simulink model "H175_Anode_Integration"  (R2023a)
settings: Solver=VariableStepAuto  StartTime=0.0  StopTime=80  RelTol=1e-3
values from neighbouring files (symbols this model uses):
  anode_tube_D = 0.01    [All_Properties.mat]    (also in anode_subsystem_parameters.m; environment_parameters.m)
  D = 0.01    [All_Properties.mat]    (also in anode_subsystem_parameters.m)
  densityHydrogen = 0.0899    [All_Properties.mat]    (also in Valve_Init.m; anode_subsystem_parameters.m)
  Kv_VL6112 = 0.8    [All_Properties.mat]    (also in anode_subsystem_parameters.m)
  N2_T = [-56.55 -50 -40 -30 -20 -10 -5 -4 -3 -2 -1 0 ... (52 elements, 1x52)]    [All_Properties.mat]    (also in anode_subsystem_parameters.m = [-56.55 -50 -40 -30 -20 -10 -5 -4 -3 -2 -1 0 1 2 3 4 5 10 20; environment_parameters.m = [-56.55, -50:10:-10, -5:1:5, 10:10:350]; stack_model_harness_parameters.m = [-56.55, -50:10:-10, -5:1:5, 10:10:350])
  p_range = 0.005    [All_Properties.mat]    (also in anode_subsystem_parameters.m)
  r_max = 0.2    [All_Properties.mat]    (also in anode_subsystem_parameters.m)
  r_min = 0.0001    [All_Properties.mat]    (also in anode_subsystem_parameters.m)
  responseTimeValve = 0.013    [All_Properties.mat]    (also in anode_subsystem_parameters.m)
libraries: fl_lib x75, nesl_utility x39, SimscapeFluids_lib x1
(part 1 of 2)
settings Model: Creator=debjani.ghosh  LastModifiedBy=adrian.taveras
settings DataIOCC: SaveFormat=StructureWithTime  ReturnWorkspaceOutputs=off  LoggingToFile=on
settings SimscapeCC: SimscapeLogType=all  SimscapeLogOpenViewer=on  SimscapeLogLimitData=off

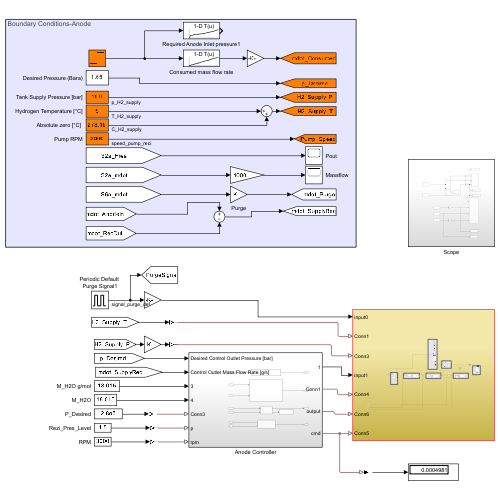
[thumbnail: Simulink's stored preview of the top-level diagram]
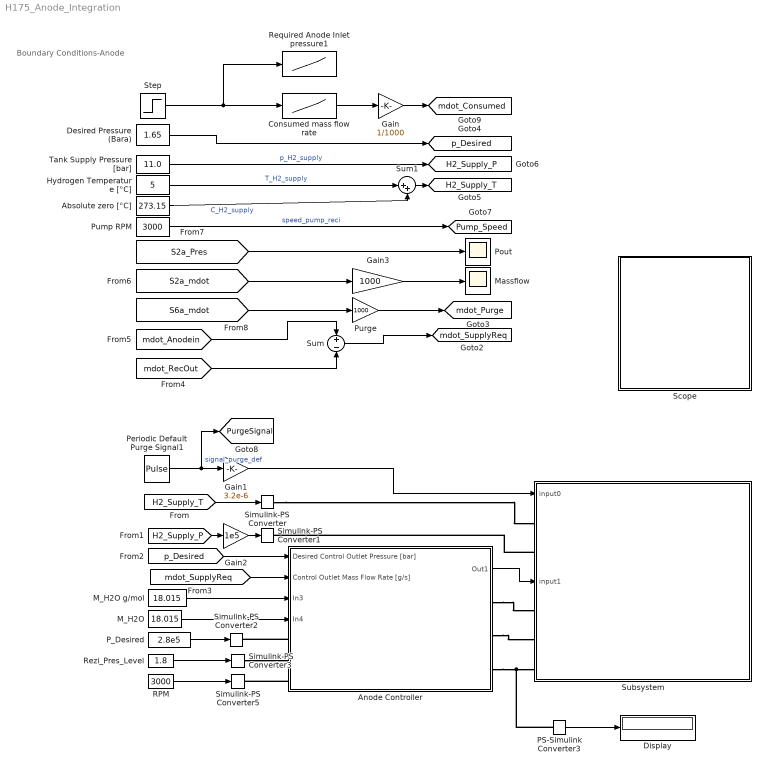
== system H175_Anode_Integration ==
  note: Boundary Conditions-Anode
  "Absolute zero [°C] " : Constant  Value=273.15
  Anode Controller : Subsystem
  Consumed mass flow rate : Lookup_n-D  NumberOfTableDimensions=1  BreakpointsForDimension1=[0;20;100;200;300;400;500;600]  Table=[0;0.1;0.5;1;1.5;2;2.5;3]  InternalRulePriority=Speed  RndMeth=Simplest
  Desired Pressure (Bara) : Constant  Value=1.65
  Display : Display
  Gain : Gain  Gain=1/1000
  Gain1 : Gain  Gain=3.2e-6
  Gain2 : Gain  Gain=1e5
  Gain3 : Gain  Gain=1000
  Hydrogen Temperature [°C] : Constant  Value=5
  M_H2O : Constant  Value=18.015
  M_H2O g/mol : Constant  Value=18.015
  Massflow : Scope
  PS-Simulink Converter3 : nesl_utility/PS-Simulink Converter  PhysicalDomain=network_engine_domain  SubClassName=ps_output  LeftPortType=input  RightPortType=output  PseudoPeriodic=off  Frequencies=[]  VectorFormat=inherit  Unit=inherit  AffineConversion=off
  P_Desired : Constant  Value=2.8e5
  Periodic Default Purge Signal1 : DiscretePulseGenerator  PulseType=Time based  Period=3  PulseWidth=5
  Pout : Scope
  Pump RPM : Constant  Value=3000
  Purge : Gain  Gain=1000
  RPM : Constant  Value=3000
  Required Anode Inlet pressure1 : Lookup_n-D  NumberOfTableDimensions=1  BreakpointsForDimension1=[0;20;100;200;300;400;500;600]  Table=[1;1.4;1.6;1.7;1.8;2;2.3;2.6]  InternalRulePriority=Speed  RndMeth=Simplest
  Rezi_Pres_Level : Constant  Value=1.8
  Scope : Subsystem
  Simulink-PS Converter : nesl_utility/Simulink-PS Converter  PhysicalDomain=network_engine_domain  SubClassName=ps_input  LeftPortType=input  RightPortType=output  PseudoPeriodic=off  Frequencies=[]  NoiseDistribution=none  NoiseParameters=[]  Unit=K  AffineConversion=off  FilteringAndDerivatives=provide  SimscapeFilterOrder=1  InputFilterTimeConstant=0.001  UdotUserProvided=0
  Simulink-PS Converter1 : nesl_utility/Simulink-PS Converter  PhysicalDomain=network_engine_domain  SubClassName=ps_input  LeftPortType=input  RightPortType=output  PseudoPeriodic=off  Frequencies=[]  NoiseDistribution=none  NoiseParameters=[]  Unit=Pa  AffineConversion=off  FilteringAndDerivatives=provide  SimscapeFilterOrder=1  InputFilterTimeConstant=0.001  UdotUserProvided=0
  Simulink-PS Converter2 : nesl_utility/Simulink-PS Converter  PhysicalDomain=network_engine_domain  SubClassName=ps_input  LeftPortType=input  RightPortType=output  PseudoPeriodic=off  Frequencies=[]  NoiseDistribution=none  NoiseParameters=[]  Unit=1  AffineConversion=off  FilteringAndDerivatives=provide  SimscapeFilterOrder=1  InputFilterTimeConstant=0.001  UdotUserProvided=0
  Simulink-PS Converter3 : nesl_utility/Simulink-PS Converter  PhysicalDomain=network_engine_domain  SubClassName=ps_input  LeftPortType=input  RightPortType=output  PseudoPeriodic=off  Frequencies=[]  NoiseDistribution=none  NoiseParameters=[]  Unit=1  AffineConversion=off  FilteringAndDerivatives=provide  SimscapeFilterOrder=1  InputFilterTimeConstant=0.001  UdotUserProvided=0
  Simulink-PS Converter5 : nesl_utility/Simulink-PS Converter  PhysicalDomain=network_engine_domain  SubClassName=ps_input  LeftPortType=input  RightPortType=output  PseudoPeriodic=off  Frequencies=[]  NoiseDistribution=none  NoiseParameters=[]  Unit=1  AffineConversion=off  FilteringAndDerivatives=provide  SimscapeFilterOrder=1  InputFilterTimeConstant=0.001  UdotUserProvided=0
  Step : Step  Time=40  Before=200  After=350  SampleTime=0
  Subsystem : Subsystem
      settings: PortSchema="{\"entries\":[{\"content\":{\"sides\":[{\"content\":{\"connectorIds\":[\"In1\",\"LConn1\",\"LConn2\",\"In2\",\"LConn3\",\"LConn4\",\"LConn5\"]},\"type\":\"ConnectorPlacement.EquallySpacedRectSide\",\"uuid\":\"6d276737-1cfb-43f0-89a6-ca57f89f04f9\"},{\"content\":{\"side\":\"RIGHT\"},\"type\":\"ConnectorPlacement.EquallySpacedRectSide\",\"uuid\":\"f7ce7b2b-f458-4a7d-a84b-f12d4a9a3d73\"},{\"content\":{\"side\":\"TOP\"},\"type\":\"ConnectorPlacement.EquallySpacedRectSide\",\"uuid\":\"f2759a84-f209-4626-aa5e-b52256180764\"}]},\"type\":\"ConnectorPlacement.EquallySpacedConnector\",\"uuid\":\"a55dce8e-c3c8-40fa-9a6a-dcd78737938e\"}],\"packageUris\":[\"http://schema.mathworks.com/mf0/Connector/R2020b\"],\"version\":\"1.0\"}"
  Sum : Sum  Inputs=+-
  Sum1 : Sum  Inputs=|++
  Tank Supply Pressure [bar] : Constant  Value=11.0
  tag scope: H2_Supply_P=global, H2_Supply_T=global, Pump_Speed=global, PurgeSignal=global, mdot_Consumed=global, mdot_Purge=global, mdot_SupplyReq=global, p_Desired=global
  wires:
  Consumed mass flow rate/1 -> Gain/1
  Hydrogen Temperature [°C]/1 -> Sum1/1  "T_H2_supply"
  "Absolute zero [°C] "/1 -> Sum1/2  "C_H2_supply"
  Sum1/1 -> [H2_Supply_T]
  Tank Supply Pressure [bar]/1 -> [H2_Supply_P]  "p_H2_supply"
  Pump RPM/1 -> [Pump_Speed]  "speed_pump_reci"
  Gain/1 -> [mdot_Consumed]
  Desired Pressure (Bara)/1 -> [p_Desired]
  Step/1 -> Required Anode Inlet pressure1/1, Consumed mass flow rate/1
  Gain2/1 -> Simulink-PS Converter1/1
  [H2_Supply_P] -> Gain2/1
  [H2_Supply_T] -> Simulink-PS Converter/1
  P_Desired/1 -> Simulink-PS Converter2/1
  Gain3/1 -> Massflow/1
  [S2a_mdot] -> Gain3/1
  [S2a_Pres] -> Pout/1
  Sum/1 -> [mdot_SupplyReq]
  [mdot_Anodein] -> Sum/1
  [mdot_RecOut] -> Sum/2
  Rezi_Pres_Level/1 -> Simulink-PS Converter3/1
  PS-Simulink Converter3/1 -> Display/1
  RPM/1 -> Simulink-PS Converter5/1
  Periodic Default Purge Signal1/1 -> Gain1/1, [PurgeSignal]  "signal_purge_def"
  Purge/1 -> [mdot_Purge]
  [S6a_mdot] -> Purge/1
  [p_Desired] -> Anode Controller/1(Desired Control Outlet Pressure [bar])
  [mdot_SupplyReq] -> Anode Controller/2(Control Outlet Mass Flow Rate [g/s])
  M_H2O g/mol/1 -> Anode Controller/3(In3)
  M_H2O/1 -> Anode Controller/4(In4)
  Gain1/1 -> Subsystem/1(input0)
  Anode Controller/1(Out1) -> Subsystem/2(input1)
  connections:
  PS-Simulink Converter3/LConn1 -- Anode Controller/RConn3 -- Subsystem/LConn5
  Anode Controller/LConn1 -- Simulink-PS Converter2/RConn1
  Simulink-PS Converter3/RConn1 -- Anode Controller/LConn2
  Anode Controller/LConn3 -- Simulink-PS Converter5/RConn1
  Simulink-PS Converter/RConn1 -- Subsystem/LConn1
  Subsystem/LConn2 -- Simulink-PS Converter1/RConn1
  Anode Controller/RConn1 -- Subsystem/LConn3
  Anode Controller/RConn2 -- Subsystem/LConn4

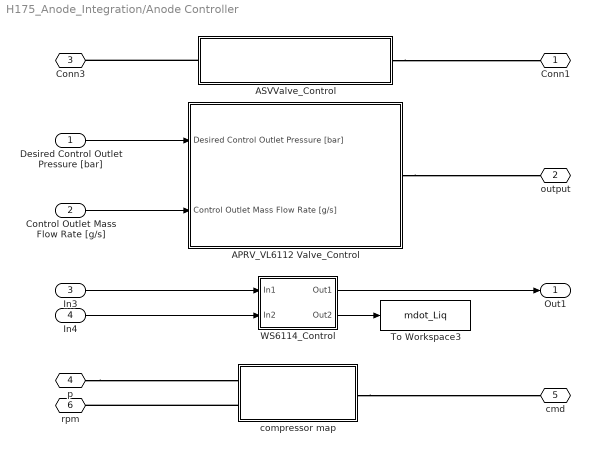
== system H175_Anode_Integration/Anode Controller ==
  Desired Control Outlet Pressure [bar] : Inport
  Control Outlet Mass Flow Rate [g/s] : Inport  Port=2
  In3 : Inport  Port=3
  In4 : Inport  Port=4
  APRV_VL6112 Valve_Control : Subsystem
  ASVValve_Control : Subsystem
  To Workspace3 : ToWorkspace  VariableName=mdot_Liq  SaveFormat=Structure With Time  SampleTime=-1
  WS6114_Control : Subsystem
  compressor map : Subsystem
  Conn1 : PMIOPort  Side=Right
  output : PMIOPort  Port=2  Side=Right
  Conn3 : PMIOPort  Port=3  Side=Left
  p : PMIOPort  Port=4  Side=Left
  cmd : PMIOPort  Port=5  Side=Right
  rpm : PMIOPort  Port=6  Side=Left
  Out1 : Outport
  wires:
  Control Outlet Mass Flow Rate [g/s]/1 -> APRV_VL6112 Valve_Control/2(Control Outlet Mass Flow Rate [g/s])
  WS6114_Control/1(Out1) -> Out1/1
  Desired Control Outlet Pressure [bar]/1 -> APRV_VL6112 Valve_Control/1(Desired Control Outlet Pressure [bar])
  WS6114_Control/2(Out2) -> To Workspace3/1
  In3/1 -> WS6114_Control/1(In1)
  In4/1 -> WS6114_Control/2(In2)
  connections:
  p/RConn1 -- compressor map/LConn1
  ASVValve_Control/RConn1 -- Conn1/RConn1
  compressor map/RConn1 -- cmd/RConn1
  ASVValve_Control/LConn1 -- Conn3/RConn1
  compressor map/LConn2 -- rpm/RConn1
  APRV_VL6112 Valve_Control/RConn1 -- output/RConn1

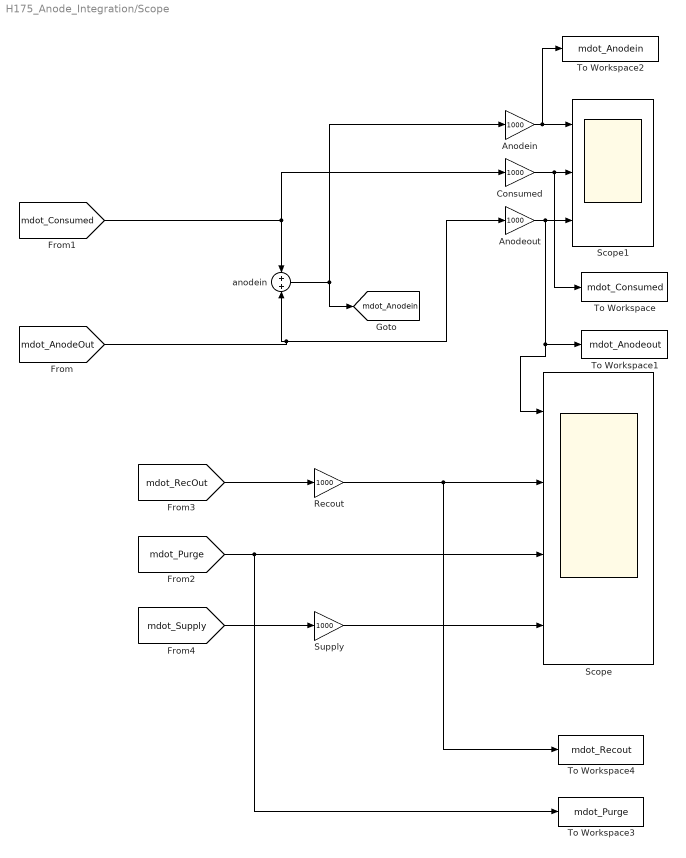
== system H175_Anode_Integration/Scope ==
  Anodein : Gain  Gain=1000
  Anodeout : Gain  Gain=1000
  Consumed : Gain  Gain=1000
  Recout : Gain  Gain=1000
  Scope : Scope  NumInputPorts=4
  Scope1 : Scope  NumInputPorts=3
  Supply : Gain  Gain=1000
  To Workspace : ToWorkspace  VariableName=mdot_Consumed  SaveFormat=Structure With Time  SampleTime=-1
  To Workspace1 : ToWorkspace  VariableName=mdot_Anodeout  SaveFormat=Structure With Time  SampleTime=-1
  To Workspace2 : ToWorkspace  VariableName=mdot_Anodein  SaveFormat=Structure With Time  SampleTime=-1
  To Workspace3 : ToWorkspace  VariableName=mdot_Purge  SaveFormat=Structure With Time  SampleTime=-1
  To Workspace4 : ToWorkspace  VariableName=mdot_Recout  SaveFormat=Structure With Time  SampleTime=-1
  anodein : Sum
  tag scope: mdot_Anodein=global
  wires:
  [mdot_Consumed] -> anodein/1, Consumed/1
  [mdot_AnodeOut] -> Anodeout/1, anodein/2
  Anodein/1 -> To Workspace2/1, Scope1/1
  Anodeout/1 -> Scope/1, To Workspace1/1, Scope1/3
  Consumed/1 -> To Workspace/1, Scope1/2
  [mdot_Purge] -> To Workspace3/1, Scope/3
  anodein/1 -> [mdot_Anodein], Anodein/1
  Recout/1 -> To Workspace4/1, Scope/2
  [mdot_RecOut] -> Recout/1
  [mdot_Supply] -> Supply/1
  Supply/1 -> Scope/4

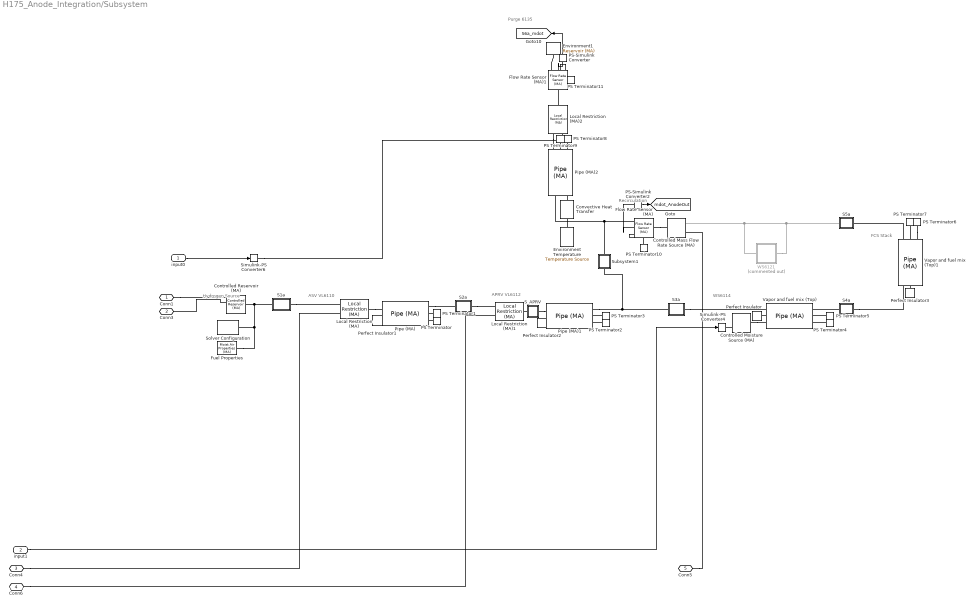
== system H175_Anode_Integration/Subsystem ==
  note: Purge 6135
  note: FCS Stack
  note: Recirculation
  note: WS6114
  note: APRV VL6112
  note: ASV VL6110
  note: Hydrogen Source
  input0 : Inport
  input1 : Inport  Port=2
  " WS6121" : Subsystem  Tag=PublishSubsystem  Commented=on
  Controlled Mass Flow Rate Source (MA) : fl_lib/Moist Air/Sources/Controlled Mass Flow Rate Source (MA)  power_spec=foundation.enum.power_spec.isentropic  area_A=pi*anode_tube_D^2/4 m^2  area_B=pi*anode_tube_D^2/4 m^2
      settings: InternalSimscapePortConfiguration="{\"Bottom\":[],\"Left\":[{\"id\":\"A\",\"label\":\"A\",\"type\":\"foundation.moist_air.moist_air\"},{\"id\":\"M\",\"label\":\"M\",\"type\":\"input\"}],\"Right\":[{\"id\":\"B\",\"label\":\"B\",\"type\":\"foundation.moist_air.moist_air\"}],\"Top\":[]}"
  Controlled Moisture Source (MA) : fl_lib/Moist Air/Sources/Moisture & Trace Gas Sources/Controlled Moisture Source (MA)  moisture_source_spec=foundation.enum.moisture_source_spec.liquid  Phi_S_specify=off  Phi_S_priority=None  Phi_S=0 kW  Phi_S_nominal_specify=off  Phi_S_nominal_unit=kW  Phi_S_nominal_value=1  mdot_w_S_specify=off  mdot_w_S_priority=None  mdot_w_S=0 kg/s  mdot_w_S_nominal_specify=off  mdot_w_S_nominal_unit=kg/s  mdot_w_S_nominal_value=1
      settings: InternalSimscapePortConfiguration="{\"Bottom\":[],\"Left\":[{\"id\":\"S\",\"label\":\"S\",\"type\":\"foundation.moist_air.moist_air_source\"}],\"Right\":[{\"id\":\"M\",\"label\":\"M\",\"type\":\"input\"},{\"id\":\"T\",\"label\":\"T\",\"type\":\"input\"}],\"Top\":[]}"
  Controlled Reservoir (MA) : fl_lib/Moist Air/Elements/Controlled Reservoir (MA)  moisture_spec=foundation.enum.moistureSpec.RelativeHumidity  trace_gas_spec=foundation.enum.trace_gas_spec.mass_fraction  RH_ws=1  area_A=0.01 m^2  input_error_spec=foundation.enum.input_range_error.warn
      settings: InternalSimscapePortConfiguration="{\"Bottom\":[],\"Left\":[{\"id\":\"A\",\"label\":\"A\",\"type\":\"foundation.moist_air.moist_air\"}],\"Right\":[{\"id\":\"T\",\"label\":\"T\",\"type\":\"input\"},{\"id\":\"P\",\"label\":\"P\",\"type\":\"input\"},{\"id\":\"W\",\"label\":\"W\",\"type\":\"input\"},{\"id\":\"G\",\"label\":\"G\",\"type\":\"input\"}],\"Top\":[]}"
  Convective Heat Transfer : fl_lib/Thermal/Thermal Elements/Convective Heat Transfer  thermal_type=foundation.enum.constant_variable.constant  area=pi*anode_tube_D*1 m^2  heat_tr_coeff=20 W/(m^2 * K)  min_heat_tr_coeff=1e-3 W/(K*m^2)  T_specify=off  T_priority=None  T=0 K  T_nominal_specify=off  T_nominal_unit=K  T_nominal_value=1  Q_specify=off  Q_priority=None  Q=0 W  Q_nominal_specify=off  Q_nominal_unit=W  Q_nominal_value=1
  Environment Temperature : fl_lib/Thermal/Thermal Sources/Temperature Source  temperature=env_T degC
  Environment1 : fl_lib/Moist Air/Elements/Reservoir (MA)  pressure_spec=foundation.enum.pressure_spec.atmospheric  reservoir_pressure=0.101325 MPa  temperature_spec=foundation.enum.temperature_spec.atmospheric  reservoir_temperature=293.15 K  moisture_spec=foundation.enum.moistureSpec.RelativeHumidity  reservoir_RH=0.5  reservoir_x_w=0.01  reservoir_y_w=0.01  reservoir_HR=0.01  reservoir_Tw=287 K  trace_gas_spec=foundation.enum.trace_gas_spec.mass_fraction  reservoir_x_g=0.001  reservoir_y_g=0.001  RH_ws=1  area_A=0.01 m^2
  Flow Rate Sensor (MA) : fl_lib/Moist Air/Sensors/Flow Rate Sensor (MA)  mass_flow_measure=true  volumetric_flow_measure=false  volumetric_flow_conditions=foundation.enum.volumetric_flow_conditions.actual  p_std=0.101325 MPa  T_std=20 degC  RH_std=0.65  energy_flow_measure=true  vapor_flow_measure=false  gas_flow_measure=false
      settings: InternalSimscapePortConfiguration="{\"Bottom\":[{\"id\":\"PHI\",\"label\":\"φ\",\"type\":\"output\"}],\"Left\":[{\"id\":\"A\",\"label\":\"A\",\"type\":\"foundation.moist_air.moist_air\"}],\"Right\":[{\"id\":\"B\",\"label\":\"B\",\"type\":\"foundation.moist_air.moist_air\"},{\"id\":\"M\",\"label\":\"M\",\"type\":\"output\"}],\"Top\":[]}"
  Flow Rate Sensor (MA)1 : fl_lib/Moist Air/Sensors/Flow Rate Sensor (MA)  mass_flow_measure=true  volumetric_flow_measure=false  volumetric_flow_conditions=foundation.enum.volumetric_flow_conditions.actual  p_std=0.101325 MPa  T_std=20 degC  RH_std=0.65  energy_flow_measure=true  vapor_flow_measure=false  gas_flow_measure=false
      settings: InternalSimscapePortConfiguration="{\"Bottom\":[{\"id\":\"PHI\",\"label\":\"φ\",\"type\":\"output\"}],\"Left\":[{\"id\":\"A\",\"label\":\"A\",\"type\":\"foundation.moist_air.moist_air\"}],\"Right\":[{\"id\":\"B\",\"label\":\"B\",\"type\":\"foundation.moist_air.moist_air\"},{\"id\":\"M\",\"label\":\"M\",\"type\":\"output\"}],\"Top\":[]}"
  Fuel Properties : fl_lib/Moist Air/Utilities/Moist Air Properties (MA)  R_a=N2_R J/kg/K  T_TLU=N2_T degC  h_a_TLU=N2_h kJ/kg  mu_a_TLU=N2_mu s*uPa  k_a_TLU=N2_k mW/m/K  p_min=1 kPa  p_max=inf MPa  T_min=min(N2_T) degC  T_max=max(N2_T) degC  properties_range_check=simscape.enum.assert.action.error  p_atm=0.101325 MPa  T_atm=20 degC  R_w=461.523 J/kg/K  p_ws_TLU=[1.71168953425982e-06; 3.93770601979424e-06; 1.28411717710344e-05; 3.80051394873809e-05; .00010323902900209; .000259873810798063; .000401741022116384; .000437454836117844; .000476040820618202; .000517704666185737; .000562664883741207; .000611212677444345; .000657088049117899; .000705987905898279; .000758082381149132; .000813549384183233; .000872574861129522; .00122818386934022; .0023392147667769; .00424668834054807; .00738442748706953; .0123512704340234; .0199458019246787; .0312006356960619; .0474147199263783; .0701823607447713; .10141797792131; .143375967241115; .198665399739302; .270259606559999; .361500961984849; .476101381081492; .618139196722055; .792053183687694; 1.0026345688121; 1.25501792086105; 1.55467186826983; 1.90739066433297; 2.31928772772542; 2.79679245576864; 3.34665187151016; 3.97593907083533; 4.69207105435535; 5.5028394740883; 6.41645928168037; 7.4416425436169; 8.58770832955728; 9.86474556030261; 11.2838558865497; 12.8575218898034; 14.6001810568052; 16.5291642526045] MPa  h_w_vap_TLU=[2836.88241275372; 2837.81392500514; 2838.63937175807; 2838.7309929628; 2838.06905313927; 2836.62597341095; 2835.60023952573; 2835.37006381376; 2835.13143158077; 2834.88429145066; 2834.62859062897; 2500.93420564316; 2498.55329907119; 2496.17495082036; 2493.79885912205; 2491.42474723191; 2489.05236104642; 2477.20875029194; 2453.54955988604; 2429.83856603313; 2406.00136954922; 2381.97406342174; 2357.69101156389; 2333.08088387814; 2308.06565480412; 2282.56034405021; 2256.47287422313; 2229.70428017508; 2202.14968030993; 2173.69998896199; 2144.24368406447; 2113.66758247452; 2081.85585110571; 2048.68725710494; 2014.03141249899; 1977.7449923284; 1939.66849592886; 1899.62342931686; 1857.40930169838; 1812.79975416601; 1765.53721731251; 1715.32525772152; 1661.81700477787; 1604.59703745016; 1543.1534616334; 1476.83692476464; 1404.80240352424; 1325.92091736114; 1238.61667822208; 1140.5102987018; 1027.62017777647; 892.733785613825] kJ/kg  h_w_TLU=[2396.55944251649; 2408.68643343608; 2427.1988031141; 2445.702165897; 2464.18429108356; 2482.62529466839; 2491.82135326629; 2493.6580151792; 2495.49372578218; 2497.32843835745; 2499.16210446923; 2500.99462758899; 2502.83092214066; 2504.6665223621; 2506.50140563013; 2508.335548891; 2510.16892865793; 2519.32352241995; 2537.56068088674; 2555.67742615292; 2573.6403223998; 2591.4109179101; 2608.9455037701; 2626.19492016262; 2643.10444358428; 2659.61377634497; 2675.58278696023; 2696.1846256545; 2716.49989553741; 2736.6235210957; 2756.61216047011; 2776.50561773853; 2796.33378922508; 2816.11979583049; 2835.88181423877; 2855.63430574511; 2875.38889327595; 2895.15500577172; 2914.94035964689; 2934.75132290228; 2954.59319330244; 2974.47041285505; 2994.38673458964; 3014.34535328009; 3034.34900867103; 3054.40006755764; 3074.50058946898; 3094.65237953784; 3114.85703128106; 3135.11596137801; 3155.43043805905; 3175.80160435813] kJ/kg  mu_w_TLU=[6.81365662228272; 7.04953750742707; 7.40970098298307; 7.76991278093907; 8.13017290129507; 8.49048134405107; 8.67065368632907; 8.70668960445667; 8.74272600580827; 8.77876289038387; 8.81480025818347; 8.85083810920707; 8.88687644345467; 8.92291526092627; 8.95895456162187; 8.99499434554147; 9.03103461268507; 9.21124319676307; 9.57169660671907; 9.93219833907507; 10.2927483938311; 10.6533467709871; 11.0139934705431; 11.3746884924991; 11.7354318368551; 12.0962235036111; 12.4570634927671; 12.8179518043231; 13.1788884382791; 13.5398733946351; 13.9009066733911; 14.2619882745471; 14.6231181981031; 14.9842964440591; 15.3455230124151; 15.7067979031711; 16.0681211163271; 16.4294926518831; 16.7909125098391; 17.1523806901951; 17.5138971929511; 17.8754620181071; 18.2370751656631; 18.5987366356191; 18.9604464279751; 19.3222045427311; 19.6840109798871; 20.0458657394431; 20.4077688213991; 20.7697202257551; 21.1317199525111; 21.4937680016671] s*uPa  k_w_TLU=[11.46288215976; 11.941997488935; 12.676358586935; 13.414208884935; 14.155548382935; 14.900377080935; 15.274099879935; 15.348949115735; 15.423833243535; 15.498752263335; 15.573706175135; 15.648694978935; 15.723718674735; 15.798777262535; 15.873870742335; 15.948999114135; 16.024162377935; 16.400502076935; 17.155798374935; 17.914583872935; 18.676858570935; 19.442622468935; 20.211875566935; 20.984617864935; 21.760849362935; 22.540570060935; 23.323779958935; 24.110479056935; 24.900667354935; 25.694344852935; 26.491511550935; 27.292167448935; 28.096312546935; 28.903946844935; 29.715070342935; 30.529683040935; 31.347784938935; 32.169376036935; 32.994456334935; 33.823025832935; 34.655084530935; 35.490632428935; 36.329669526935; 37.172195824935; 38.018211322935; 38.867716020935; 39.720709918935; 40.577193016935; 41.437165314935; 42.300626812935; 43.167577510935; 44.038017408935] mW/m/K  D_w=25 mm^2/s  trace_gas_model=foundation.enum.trace_gas_model.track_properties  R_g=H2_R J/kg/K  h_g_TLU=H2_h kJ/kg  mu_g_TLU=H2_mu s*uPa  k_g_TLU=H2_k mW/m/K  D_g=H2_D mm^2/s
      settings: AttributesFormatString=|
      | dry air --> N2
      | water vapor --> H2O
      | trace gas --> H2
  Local Restriction (MA) : fl_lib/Moist Air/Elements/Local Restriction (MA)  restriction_type=foundation.enum.restriction_type.variable  restriction_area=0.005 m^2  min_area=0.00001e-6 m^2  max_area=4.75e-6 m^2  area=0.00358 m^2  Cd=0.80  B_lam=0.999
      settings: LogSimulationData=on
  Local Restriction (MA)1 : fl_lib/Moist Air/Elements/Local Restriction (MA)  restriction_type=foundation.enum.restriction_type.variable  restriction_area=0.005 m^2  min_area=0.00001e-6 m^2  max_area=4.75e-6 m^2  area=0.00358 m^2  Cd=0.80  B_lam=0.999
      settings: LogSimulationData=on
  Local Restriction (MA)2 : fl_lib/Moist Air/Elements/Local Restriction (MA)  restriction_type=foundation.enum.restriction_type.variable  restriction_area=0.005 m^2  min_area=0.00001e-6 m^2  max_area=3.2e-6 m^2  area=0.00358 m^2  Cd=0.80  B_lam=0.999
      settings: LogSimulationData=on
  PS Terminator{,1..11} (12 alike) : fl_lib/Physical Signals/Sinks/PS Terminator
  PS-Simulink Converter : nesl_utility/PS-Simulink Converter  PhysicalDomain=network_engine_domain  SubClassName=ps_output  LeftPortType=input  RightPortType=output  PseudoPeriodic=off  Frequencies=[]  VectorFormat=inherit  Unit=inherit  AffineConversion=off
  PS-Simulink Converter2 : nesl_utility/PS-Simulink Converter  PhysicalDomain=network_engine_domain  SubClassName=ps_output  LeftPortType=input  RightPortType=output  PseudoPeriodic=off  Frequencies=[]  VectorFormat=inherit  Unit=inherit  AffineConversion=off
  Perfect Insulator{,1..3} (4 alike) : fl_lib/Thermal/Thermal Elements/Perfect Insulator  T_specify=off  T_priority=None  T=0 K  T_nominal_specify=off  T_nominal_unit=K  T_nominal_value=1
  Pipe (MA) : fl_lib/Moist Air/Elements/Pipe (MA)  length=1 m  area=pi*anode_tube_D^2/4 m^2  Dh=anode_tube_D m  length_add=0.1 m  roughness=15e-6 m  Re_lam=2000  Re_tur=4000  shape_factor=64  Nu_lam=3.66  wall_condensation=simscape.enum.onoff.off  RH_ws=1  time_constant=1e-3 s  moisture_trace_gas_source=foundation.enum.moisture_trace_gas_source.none  moisture_source_spec=foundation.enum.moisture_source_spec.vapor  moisture_mass_flow=0 kg/s  moisture_temperature_spec=foundation.enum.temperature_spec.atmospheric  moisture_temperature=293.15 K  trace_gas_mass_flow=0 kg/s  trace_gas_temperature_spec=foundation.enum.temperature_spec.atmospheric  trace_gas_temperature=293.15 K  p_I_specify=on  p_I_priority=High  p_I=env_p MPa  p_I_nominal_specify=off  p_I_nominal_unit=MPa  p_I_nominal_value=1  T_I_specify=on  T_I_priority=High  T_I=env_T degC  T_I_nominal_specify=off  T_I_nominal_unit=K  T_I_nominal_value=1  RH_I_specify=off  RH_I_priority=High  RH_I=0  RH_I_nominal_specify=off  RH_I_nominal_unit=1  RH_I_nominal_value=1  x_w_I_specify=off  x_w_I_priority=None  x_w_I=0  x_w_I_nominal_specify=off  x_w_I_nominal_unit=1  x_w_I_nominal_value=1  y_w_I_specify=off  y_w_I_priority=None  y_w_I=0  y_w_I_nominal_specify=off  y_w_I_nominal_unit=1  y_w_I_nominal_value=1  HR_I_specify=off  HR_I_priority=None  HR_I=0  HR_I_nominal_specify=off  HR_I_nominal_unit=1  HR_I_nominal_value=1  x_g_I_specify=on  x_g_I_priority=None  x_g_I=0  x_g_I_nominal_specify=off  x_g_I_nominal_unit=1  x_g_I_nominal_value=1  y_g_I_specify=on  y_g_I_priority=High  y_g_I=tank_yH2  y_g_I_nominal_specify=off  y_g_I_nominal_unit=1  y_g_I_nominal_value=1
  Pipe (MA)1 : fl_lib/Moist Air/Elements/Pipe (MA)  length=1 m  area=pi*anode_tube_D^2/4 m^2  Dh=anode_tube_D m  length_add=0.1 m  roughness=15e-6 m  Re_lam=2000  Re_tur=4000  shape_factor=64  Nu_lam=3.66  wall_condensation=simscape.enum.onoff.off  RH_ws=1  time_constant=1e-3 s  moisture_trace_gas_source=foundation.enum.moisture_trace_gas_source.none  moisture_source_spec=foundation.enum.moisture_source_spec.vapor  moisture_mass_flow=0 kg/s  moisture_temperature_spec=foundation.enum.temperature_spec.atmospheric  moisture_temperature=293.15 K  trace_gas_mass_flow=0 kg/s  trace_gas_temperature_spec=foundation.enum.temperature_spec.atmospheric  trace_gas_temperature=293.15 K  p_I_specify=on  p_I_priority=High  p_I=env_p MPa  p_I_nominal_specify=off  p_I_nominal_unit=MPa  p_I_nominal_value=1  T_I_specify=on  T_I_priority=High  T_I=env_T degC  T_I_nominal_specify=off  T_I_nominal_unit=K  T_I_nominal_value=1  RH_I_specify=off  RH_I_priority=High  RH_I=0  RH_I_nominal_specify=off  RH_I_nominal_unit=1  RH_I_nominal_value=1  x_w_I_specify=off  x_w_I_priority=None  x_w_I=0  x_w_I_nominal_specify=off  x_w_I_nominal_unit=1  x_w_I_nominal_value=1  y_w_I_specify=off  y_w_I_priority=None  y_w_I=0  y_w_I_nominal_specify=off  y_w_I_nominal_unit=1  y_w_I_nominal_value=1  HR_I_specify=off  HR_I_priority=None  HR_I=0  HR_I_nominal_specify=off  HR_I_nominal_unit=1  HR_I_nominal_value=1  x_g_I_specify=on  x_g_I_priority=None  x_g_I=0  x_g_I_nominal_specify=off  x_g_I_nominal_unit=1  x_g_I_nominal_value=1  y_g_I_specify=on  y_g_I_priority=High  y_g_I=tank_yH2  y_g_I_nominal_specify=off  y_g_I_nominal_unit=1  y_g_I_nominal_value=1
  Pipe (MA)2 : fl_lib/Moist Air/Elements/Pipe (MA)  length=1 m  area=pi*anode_tube_D^2/4 m^2  Dh=anode_tube_D m  length_add=0.1 m  roughness=15e-6 m  Re_lam=2000  Re_tur=4000  shape_factor=64  Nu_lam=3.66  wall_condensation=simscape.enum.onoff.off  RH_ws=1  time_constant=1e-3 s  moisture_trace_gas_source=foundation.enum.moisture_trace_gas_source.none  moisture_source_spec=foundation.enum.moisture_source_spec.vapor  moisture_mass_flow=0 kg/s  moisture_temperature_spec=foundation.enum.temperature_spec.atmospheric  moisture_temperature=293.15 K  trace_gas_mass_flow=0 kg/s  trace_gas_temperature_spec=foundation.enum.temperature_spec.atmospheric  trace_gas_temperature=293.15 K  p_I_specify=on  p_I_priority=High  p_I=env_p MPa  p_I_nominal_specify=off  p_I_nominal_unit=MPa  p_I_nominal_value=1  T_I_specify=on  T_I_priority=High  T_I=env_T degC  T_I_nominal_specify=off  T_I_nominal_unit=K  T_I_nominal_value=1  RH_I_specify=off  RH_I_priority=High  RH_I=0  RH_I_nominal_specify=off  RH_I_nominal_unit=1  RH_I_nominal_value=1  x_w_I_specify=off  x_w_I_priority=None  x_w_I=0  x_w_I_nominal_specify=off  x_w_I_nominal_unit=1  x_w_I_nominal_value=1  y_w_I_specify=off  y_w_I_priority=None  y_w_I=0  y_w_I_nominal_specify=off  y_w_I_nominal_unit=1  y_w_I_nominal_value=1  HR_I_specify=off  HR_I_priority=None  HR_I=0  HR_I_nominal_specify=off  HR_I_nominal_unit=1  HR_I_nominal_value=1  x_g_I_specify=on  x_g_I_priority=None  x_g_I=0  x_g_I_nominal_specify=off  x_g_I_nominal_unit=1  x_g_I_nominal_value=1  y_g_I_specify=on  y_g_I_priority=High  y_g_I=tank_yH2  y_g_I_nominal_specify=off  y_g_I_nominal_unit=1  y_g_I_nominal_value=1
  S1a : Subsystem
  S2a : Subsystem
  S3a : Subsystem
  S4a : Subsystem
  S5a : Subsystem  Tag=PublishSubsystem
  S_APRV : Subsystem
  Simulink-PS Converter4 : nesl_utility/Simulink-PS Converter  PhysicalDomain=network_engine_domain  SubClassName=ps_input  LeftPortType=input  RightPortType=output  PseudoPeriodic=off  Frequencies=[]  NoiseDistribution=none  NoiseParameters=[]  Unit=1  AffineConversion=off  FilteringAndDerivatives=provide  SimscapeFilterOrder=1  InputFilterTimeConstant=0.001  UdotUserProvided=0
  Simulink-PS Converter6 : nesl_utility/Simulink-PS Converter  PhysicalDomain=network_engine_domain  SubClassName=ps_input  LeftPortType=input  RightPortType=output  PseudoPeriodic=off  Frequencies=[]  NoiseDistribution=none  NoiseParameters=[]  Unit=1  AffineConversion=off  FilteringAndDerivatives=provide  SimscapeFilterOrder=1  InputFilterTimeConstant=0.001  UdotUserProvided=0
  Solver Configuration : nesl_utility/Solver Configuration  PhysicalDomain=network_engine_domain  SubClassName=solver  LeftPortType=input  RightPortType=generic  Tones=[]  Harmonics=[]  SimulateNoise=off  Profile=off  UseLocalSampling=off  EnableSwitchedLinearOptims=on  FrequencyDomain=off  UseCCode=off  RelTol=0.001  AbsTol=0.001  MinStep=1e-09  ToWorkspace=off  RevertToSquareIcSolve=off  NumHomotopyIterations=100  PhasorMode=off  PhasorModeNumHarmonics=1  ConsistencySolver=NEWTON_XTOL_AFTER_FTOL  IndexReductionMethod=DerivativeReplacement  DoDC=off  ResidualTolerance=1e-09  ConsistencyTolSource=GLOBAL  ConsistencyAbsTol=0.001  ConsistencyRelTol=0.001  ConsistencyTolFactor=0.001  UseLocalSolver=off  LocalSolverChoice=NE_BACKWARD_EULER_ADVANCER  ResolveIndetEquations=on  FunctionEvalNumThread=1  LocalSolverSampleTime=0.001  DoFixedCost=off  MaxNonlinIter=3  MaxModeIter=2  ComputeImpulses=off  ImpulseIterations=2  LinearAlgebra=auto  LinearAlgebraNumThread=0  EquationFormulation=NE_TIME_EF  DelaysMemoryBudget=1024  AutomaticFiltering=on  FilteringTimeConstant=0.001  PartitionStorageMethod=AS_NEEDED  PartitionMemoryBudget=1024  PartitionMethod=ROBUST
  Subsystem1 : Subsystem
  Vapor and fuel mix (Top) : fl_lib/Moist Air/Elements/Pipe (MA)  length=0.25 m  area=pi*0.05^2/4 m^2  Dh=0.05 m  length_add=0.1 m  roughness=15e-6 m  Re_lam=2000  Re_tur=4000  shape_factor=64  Nu_lam=3.66  wall_condensation=simscape.enum.onoff.off  RH_ws=1  time_constant=1e-3 s  moisture_trace_gas_source=foundation.enum.moisture_trace_gas_source.controlled  moisture_source_spec=foundation.enum.moisture_source_spec.vapor  moisture_mass_flow=0 kg/s  moisture_temperature_spec=foundation.enum.temperature_spec.atmospheric  moisture_temperature=293.15 K  trace_gas_mass_flow=0 kg/s  trace_gas_temperature_spec=foundation.enum.temperature_spec.atmospheric  trace_gas_temperature=293.15 K  p_I_specify=on  p_I_priority=High  p_I=env_p MPa  p_I_nominal_specify=off  p_I_nominal_unit=MPa  p_I_nominal_value=1  T_I_specify=on  T_I_priority=High  T_I=env_T degC  T_I_nominal_specify=off  T_I_nominal_unit=K  T_I_nominal_value=1  RH_I_specify=off  RH_I_priority=High  RH_I=0  RH_I_nominal_specify=off  RH_I_nominal_unit=1  RH_I_nominal_value=1  x_w_I_specify=off  x_w_I_priority=None  x_w_I=0  x_w_I_nominal_specify=off  x_w_I_nominal_unit=1  x_w_I_nominal_value=1  y_w_I_specify=off  y_w_I_priority=None  y_w_I=0  y_w_I_nominal_specify=off  y_w_I_nominal_unit=1  y_w_I_nominal_value=1  HR_I_specify=off  HR_I_priority=None  HR_I=0  HR_I_nominal_specify=off  HR_I_nominal_unit=1  HR_I_nominal_value=1  x_g_I_specify=on  x_g_I_priority=None  x_g_I=0  x_g_I_nominal_specify=off  x_g_I_nominal_unit=1  x_g_I_nominal_value=1  y_g_I_specify=on  y_g_I_priority=High  y_g_I=tank_yH2  y_g_I_nominal_specify=off  y_g_I_nominal_unit=1  y_g_I_nominal_value=1
      settings: InternalSimscapePortConfiguration="{\"Bottom\":[],\"Left\":[{\"id\":\"A\",\"label\":\"A\",\"type\":\"foundation.moist_air.moist_air\"},{\"id\":\"H\",\"label\":\"H\",\"type\":\"foundation.thermal.thermal\"},{\"id\":\"S\",\"label\":\"S\",\"type\":\"foundation.moist_air.moist_air_source\"}],\"Right\":[{\"id\":\"B\",\"label\":\"B\",\"type\":\"foundation.moist_air.moist_air\"},{\"id\":\"W\",\"label\":\"W\",\"type\":\"output\"},{\"id\":\"F\",\"label\":\"F\",\"type\":\"output\"}],\"Top\":[]}"
  Vapor and fuel mix (Top)1 : fl_lib/Moist Air/Elements/Pipe (MA)  length=0.25 m  area=pi*0.05^2/4 m^2  Dh=0.05 m  length_add=0.1 m  roughness=15e-6 m  Re_lam=2000  Re_tur=4000  shape_factor=64  Nu_lam=3.66  wall_condensation=simscape.enum.onoff.off  RH_ws=1  time_constant=1e-3 s  moisture_trace_gas_source=foundation.enum.moisture_trace_gas_source.controlled  moisture_source_spec=foundation.enum.moisture_source_spec.vapor  moisture_mass_flow=0 kg/s  moisture_temperature_spec=foundation.enum.temperature_spec.atmospheric  moisture_temperature=293.15 K  trace_gas_mass_flow=0 kg/s  trace_gas_temperature_spec=foundation.enum.temperature_spec.atmospheric  trace_gas_temperature=293.15 K  p_I_specify=on  p_I_priority=High  p_I=env_p MPa  p_I_nominal_specify=off  p_I_nominal_unit=MPa  p_I_nominal_value=1  T_I_specify=on  T_I_priority=High  T_I=env_T degC  T_I_nominal_specify=off  T_I_nominal_unit=K  T_I_nominal_value=1  RH_I_specify=off  RH_I_priority=High  RH_I=0  RH_I_nominal_specify=off  RH_I_nominal_unit=1  RH_I_nominal_value=1  x_w_I_specify=off  x_w_I_priority=None  x_w_I=0  x_w_I_nominal_specify=off  x_w_I_nominal_unit=1  x_w_I_nominal_value=1  y_w_I_specify=off  y_w_I_priority=None  y_w_I=0  y_w_I_nominal_specify=off  y_w_I_nominal_unit=1  y_w_I_nominal_value=1  HR_I_specify=off  HR_I_priority=None  HR_I=0  HR_I_nominal_specify=off  HR_I_nominal_unit=1  HR_I_nominal_value=1  x_g_I_specify=on  x_g_I_priority=None  x_g_I=0  x_g_I_nominal_specify=off  x_g_I_nominal_unit=1  x_g_I_nominal_value=1  y_g_I_specify=on  y_g_I_priority=High  y_g_I=tank_yH2  y_g_I_nominal_specify=off  y_g_I_nominal_unit=1  y_g_I_nominal_value=1
      settings: InternalSimscapePortConfiguration="{\"Bottom\":[],\"Left\":[{\"id\":\"A\",\"label\":\"A\",\"type\":\"foundation.moist_air.moist_air\"},{\"id\":\"H\",\"label\":\"H\",\"type\":\"foundation.thermal.thermal\"},{\"id\":\"S\",\"label\":\"S\",\"type\":\"foundation.moist_air.moist_air_source\"}],\"Right\":[{\"id\":\"B\",\"label\":\"B\",\"type\":\"foundation.moist_air.moist_air\"},{\"id\":\"W\",\"label\":\"W\",\"type\":\"output\"},{\"id\":\"F\",\"label\":\"F\",\"type\":\"output\"}],\"Top\":[]}"
  Conn1 : PMIOPort  Side=Left
  Conn3 : PMIOPort  Port=2  Side=Left
  Conn4 : PMIOPort  Port=3  Side=Left
  Conn6 : PMIOPort  Port=4  Side=Left
  Conn5 : PMIOPort  Port=5  Side=Left
  tag scope: S6a_mdot=global, mdot_AnodeOut=global
  wires:
  input1/1 -> Simulink-PS Converter4/1
  PS-Simulink Converter/1 -> [S6a_mdot]
  PS-Simulink Converter2/1 -> [mdot_AnodeOut]
  input0/1 -> Simulink-PS Converter6/1
  connections:
  Local Restriction (MA)2/RConn1 -- Flow Rate Sensor (MA)1/LConn1
  Simulink-PS Converter4/RConn1 -- Controlled Moisture Source (MA)/RConn1
  Vapor and fuel mix (Top)1/RConn1 -- S5a/RConn1
  Controlled Moisture Source (MA)/LConn1 -- Vapor and fuel mix (Top)/LConn3
  Vapor and fuel mix (Top)1/RConn2 -- PS Terminator7/LConn1
  PS Terminator6/LConn1 -- Vapor and fuel mix (Top)1/RConn3
  PS Terminator10/LConn1 -- Flow Rate Sensor (MA)/RConn3
  S3a/RConn1 -- Vapor and fuel mix (Top)/LConn1
  PS Terminator2/LConn1 -- Pipe (MA)1/RConn3
  " WS6121"/LConn1 -- " WS6121"/RConn1 -- Controlled Mass Flow Rate Source (MA)/LConn1 -- S5a/LConn1
  Controlled Reservoir (MA)/RConn2 -- Conn3/RConn1
  Perfect Insulator/LConn1 -- Vapor and fuel mix (Top)/LConn2
  PS-Simulink Converter2/LConn1 -- Flow Rate Sensor (MA)/RConn2
  PS Terminator3/LConn1 -- Pipe (MA)1/RConn2
  Pipe (MA)/RConn1 -- S2a/LConn1
  S_APRV/RConn1 -- Pipe (MA)1/LConn1
  Pipe (MA)2/RConn2 -- PS Terminator9/LConn1
  Pipe (MA)1/RConn1 -- S3a/LConn1 -- Subsystem1/LConn1
  PS Terminator5/LConn1 -- Vapor and fuel mix (Top)/RConn2
  S4a/LConn1 -- Vapor and fuel mix (Top)/RConn1
  PS Terminator11/LConn1 -- Flow Rate Sensor (MA)1/RConn3
  Fuel Properties/RConn1 -- S1a/LConn1 -- Controlled Reservoir (MA)/LConn1 -- Solver Configuration/RConn1
  Local Restriction (MA)/RConn1 -- Pipe (MA)/LConn1
  S1a/RConn1 -- Local Restriction (MA)/LConn1
  Flow Rate Sensor (MA)/RConn1 -- Pipe (MA)2/LConn1 -- Subsystem1/RConn1
  Perfect Insulator3/LConn1 -- Vapor and fuel mix (Top)1/LConn2
  Pipe (MA)2/RConn3 -- PS Terminator8/LConn1
  PS Terminator1/LConn1 -- Pipe (MA)/RConn2
  Environment Temperature/LConn1 -- Convective Heat Transfer/RConn1
  Conn5/RConn1 -- Controlled Mass Flow Rate Source (MA)/LConn2
  Local Restriction (MA)2/LConn1 -- Pipe (MA)2/RConn1
  Flow Rate Sensor (MA)1/RConn1 -- Environment1/LConn1
  Pipe (MA)/LConn2 -- Perfect Insulator1/LConn1
  PS Terminator/LConn1 -- Pipe (MA)/RConn3
  Conn1/RConn1 -- Controlled Reservoir (MA)/RConn1
  Flow Rate Sensor (MA)/LConn1 -- Controlled Mass Flow Rate Source (MA)/RConn1
  Local Restriction (MA)1/RConn1 -- S_APRV/LConn1
  S4a/RConn1 -- Vapor and fuel mix (Top)1/LConn1
  Flow Rate Sensor (MA)1/RConn2 -- PS-Simulink Converter/LConn1
  Convective Heat Transfer/LConn1 -- Pipe (MA)2/LConn2
  Conn6/RConn1 -- Local Restriction (MA)1/LConn2
  PS Terminator4/LConn1 -- Vapor and fuel mix (Top)/RConn3
  Perfect Insulator2/LConn1 -- Pipe (MA)1/LConn2
  S2a/RConn1 -- Local Restriction (MA)1/LConn1
  Simulink-PS Converter6/RConn1 -- Local Restriction (MA)2/LConn2
  Conn4/RConn1 -- Local Restriction (MA)/LConn2

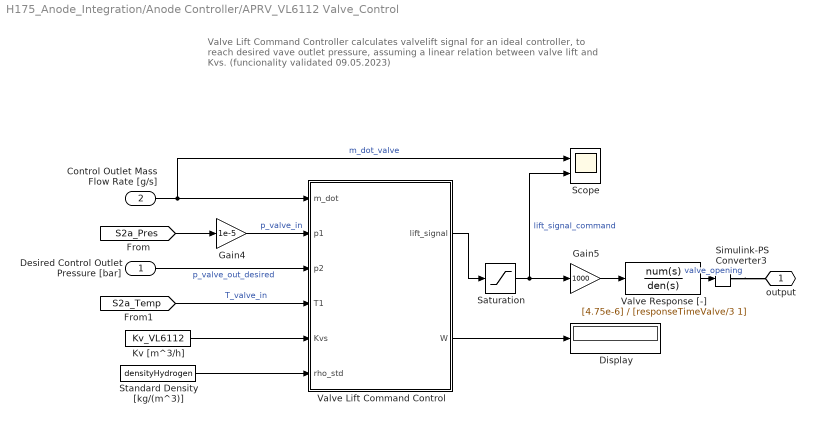
== system H175_Anode_Integration/Anode Controller/APRV_VL6112 Valve_Control ==
  note: Valve Lift Command Controller calculates valvelift signal for an
      | ideal controller, to reach desired vave outlet pressure, assuming
      | a linear relation between valve lift and Kvs.
      | (funcionality validated 09.05.2023)
  Desired Control Outlet Pressure [bar] : Inport
  Control Outlet Mass Flow Rate [g/s] : Inport  Port=2
  Display : Display
  Gain4 : Gain  Gain=1e-5
  Gain5 : Gain  Gain=1000
  Kv [m^3/h] : Constant  Value=Kv_VL6112
  Saturation : Saturate  UpperLimit=1  LowerLimit=0
  Scope : Scope  NumInputPorts=2
  Simulink-PS Converter3 : nesl_utility/Simulink-PS Converter  PhysicalDomain=network_engine_domain  SubClassName=ps_input  LeftPortType=input  RightPortType=output  PseudoPeriodic=off  Frequencies=[]  NoiseDistribution=none  NoiseParameters=[]  Unit=m^2  AffineConversion=off  FilteringAndDerivatives=provide  SimscapeFilterOrder=1  InputFilterTimeConstant=0.001  UdotUserProvided=0
  Standard Density [kg/(m^3)] : Constant  Value=densityHydrogen
  Valve Lift Command Control : MATLAB Function  TreatAsAtomicUnit=on
  Valve Response [-] : TransferFcn  Numerator=[4.75e-6]  Denominator=[responseTimeValve/3 1]
  output : PMIOPort  Side=Right
  wires:
  [S2a_Pres] -> Gain4/1
  Valve Response [-]/1 -> Simulink-PS Converter3/1  "valve_opening"
  Gain5/1 -> Valve Response [-]/1
  Valve Lift Command Control/2(W) -> Display/1
  Saturation/1 -> Gain5/1, Scope/2  "lift_signal_command"
  Valve Lift Command Control/1(lift_signal) -> Saturation/1
  Standard Density [kg/(m^3)]/1 -> Valve Lift Command Control/6(rho_std)
  Kv [m^3/h]/1 -> Valve Lift Command Control/5(Kvs)
  [S2a_Temp] -> Valve Lift Command Control/4(T1)  "T_valve_in"
  Control Outlet Mass Flow Rate [g/s]/1 -> Valve Lift Command Control/1(m_dot), Scope/1  "m_dot_valve"
  Gain4/1 -> Valve Lift Command Control/2(p1)  "p_valve_in"
  Desired Control Outlet Pressure [bar]/1 -> Valve Lift Command Control/3(p2)  "p_valve_out_desired"
  connections:
  Simulink-PS Converter3/RConn1 -- output/RConn1

== system H175_Anode_Integration/Anode Controller/ASVValve_Control ==
  PS Add : fl_lib/Physical Signals/Functions/PS Add
  PS Constant : fl_lib/Physical Signals/Sources/PS Constant  constant=r_max^2
  PS Gain : fl_lib/Physical Signals/Functions/PS Gain  gain=(r_min^2 - r_max^2)/p_range
  PS Gain1 : fl_lib/Physical Signals/Functions/PS Gain  gain=pi*D^2/4 m^2
  PS Subtract : fl_lib/Physical Signals/Functions/PS Subtract
  Pa to MPa : fl_lib/Physical Signals/Functions/PS Gain  gain=.000001
  Simulink-PS Converter : nesl_utility/Simulink-PS Converter  PhysicalDomain=network_engine_domain  SubClassName=ps_input  LeftPortType=input  RightPortType=output  PseudoPeriodic=off  Frequencies=[]  NoiseDistribution=none  NoiseParameters=[]  Unit=1  AffineConversion=off  FilteringAndDerivatives=provide  SimscapeFilterOrder=1  InputFilterTimeConstant=0.001  UdotUserProvided=0
  Conn3 : PMIOPort  Side=Left
  Conn1 : PMIOPort  Port=2  Side=Right
  wires:
  [S2a_Pres] -> Simulink-PS Converter/1
  connections:
  PS Gain1/RConn1 -- Conn1/RConn1
  PS Add/RConn1 -- PS Gain1/LConn1
  PS Constant/RConn1 -- PS Add/LConn1
  PS Subtract/LConn2 -- Conn3/RConn1
  PS Gain/LConn1 -- Pa to MPa/RConn1
  PS Add/LConn2 -- PS Gain/RConn1
  Simulink-PS Converter/RConn1 -- PS Subtract/LConn1
  Pa to MPa/LConn1 -- PS Subtract/RConn1

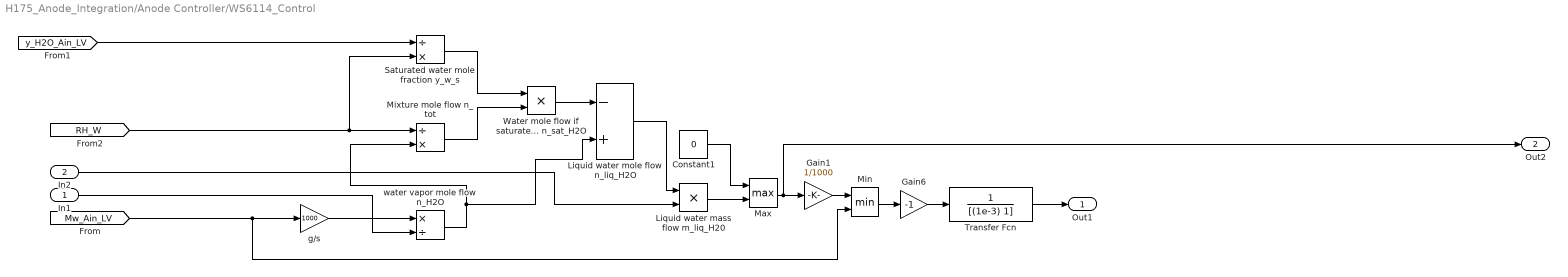
== system H175_Anode_Integration/Anode Controller/WS6114_Control ==
  In1 : Inport
  In2 : Inport  Port=2
  Constant1 : Constant  Value=0
  Gain1 : Gain  Gain=1/1000
  Gain6 : Gain  Gain=-1
  Liquid water mass flow m_liq_H20 : Product
  Liquid water mole flow n_liq_H2O : Sum  Inputs=-+
  Max : MinMax  Function=max  Inputs=2
  Min : MinMax  Inputs=2
  Mixture mole flow n_tot : Product  Inputs=/*
  Saturated water mole fraction y_w_s : Product  Inputs=/*
  Transfer Fcn : TransferFcn  Denominator=[(1e-3) 1]
  Water mole flow if saturated n_sat_H2O : Product
  g/s : Gain  Gain=1000
  water vapor mole flow n_H2O : Product  Inputs=*/
  Out1 : Outport
  Out2 : Outport  Port=2
  wires:
  Max/1 -> Out2/1, Gain1/1
  [Mw_Ain_LV] -> Min/2, g/s/1
  water vapor mole flow n_H2O/1 -> Mixture mole flow n_tot/2, Liquid water mole flow n_liq_H2O/2
  Min/1 -> Gain6/1
  Constant1/1 -> Max/1
  In1/1 -> water vapor mole flow n_H2O/2
  g/s/1 -> water vapor mole flow n_H2O/1
  Liquid water mole flow n_liq_H2O/1 -> Liquid water mass flow m_liq_H20/1
  In2/1 -> Liquid water mass flow m_liq_H20/2
  Gain1/1 -> Min/1
  Gain6/1 -> Transfer Fcn/1
  Mixture mole flow n_tot/1 -> Water mole flow if saturated n_sat_H2O/2
  Liquid water mass flow m_liq_H20/1 -> Max/2
  Water mole flow if saturated n_sat_H2O/1 -> Liquid water mole flow n_liq_H2O/1
  [RH_W] -> Mixture mole flow n_tot/1, Saturated water mole fraction y_w_s/2
  Transfer Fcn/1 -> Out1/1
  [y_H2O_Ain_LV] -> Saturated water mole fraction y_w_s/1
  Saturated water mole fraction y_w_s/1 -> Water mole flow if saturated n_sat_H2O/1

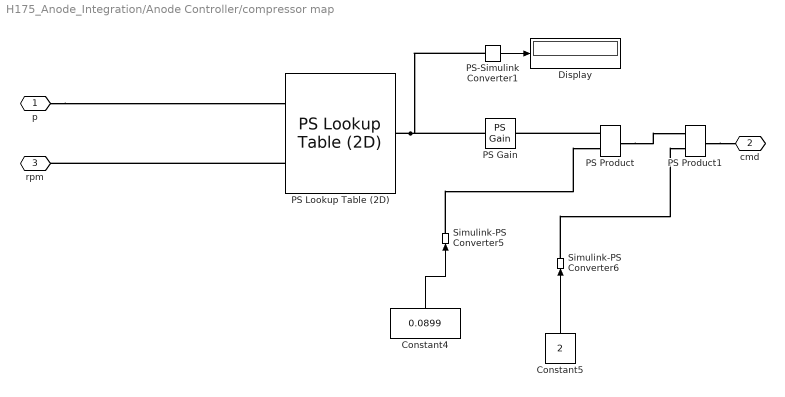
== system H175_Anode_Integration/Anode Controller/compressor map ==
  Constant4 : Constant  Value=0.0899
  Constant5 : Constant  Value=2
  Display : Display
  PS Gain : fl_lib/Physical Signals/Functions/PS Gain  gain=1/3600
  PS Lookup Table (2D) : fl_lib/Physical Signals/Lookup Tables/PS Lookup Table (2D)  x1=comp6122_p_out  x2=comp6122_rpm  f=comp6122_V_dot  interp_method=simscape.enum.interpolation.linear  extrap_method=simscape.enum.extrapolation.linear
  PS Product : fl_lib/Physical Signals/Functions/PS Product
  PS Product1 : fl_lib/Physical Signals/Functions/PS Product
  PS-Simulink Converter1 : nesl_utility/PS-Simulink Converter  PhysicalDomain=network_engine_domain  SubClassName=ps_output  LeftPortType=input  RightPortType=output  PseudoPeriodic=off  Frequencies=[]  VectorFormat=inherit  Unit=inherit  AffineConversion=off
  Simulink-PS Converter5 : nesl_utility/Simulink-PS Converter  PhysicalDomain=network_engine_domain  SubClassName=ps_input  LeftPortType=input  RightPortType=output  PseudoPeriodic=off  Frequencies=[]  NoiseDistribution=none  NoiseParameters=[]  Unit=1  AffineConversion=on  FilteringAndDerivatives=provide  SimscapeFilterOrder=1  InputFilterTimeConstant=0.001  UdotUserProvided=0
  Simulink-PS Converter6 : nesl_utility/Simulink-PS Converter  PhysicalDomain=network_engine_domain  SubClassName=ps_input  LeftPortType=input  RightPortType=output  PseudoPeriodic=off  Frequencies=[]  NoiseDistribution=none  NoiseParameters=[]  Unit=1  AffineConversion=on  FilteringAndDerivatives=provide  SimscapeFilterOrder=1  InputFilterTimeConstant=0.001  UdotUserProvided=0
  p : PMIOPort  Side=Left
  cmd : PMIOPort  Port=2  Side=Right
  rpm : PMIOPort  Port=3  Side=Left
  wires:
  Constant4/1 -> Simulink-PS Converter5/1
  Constant5/1 -> Simulink-PS Converter6/1
  PS-Simulink Converter1/1 -> Display/1
  connections:
  Simulink-PS Converter5/RConn1 -- PS Product/LConn2
  PS Lookup Table (2D)/RConn1 -- PS Gain/LConn1 -- PS-Simulink Converter1/LConn1
  PS Product/RConn1 -- PS Product1/LConn1
  PS Product/LConn1 -- PS Gain/RConn1
  PS Lookup Table (2D)/LConn2 -- rpm/RConn1
  Simulink-PS Converter6/RConn1 -- PS Product1/LConn2
  PS Product1/RConn1 -- cmd/RConn1
  p/RConn1 -- PS Lookup Table (2D)/LConn1
